simulink model "model"  (R2020b)
settings: Solver=VariableStepAuto  StartTime=0.0  StopTime=10.0  MaxStep=0.001  RelTol=1e-3
settings Model: Creator=Vrunda M Balgi  LastModifiedBy=Vrunda M Balgi

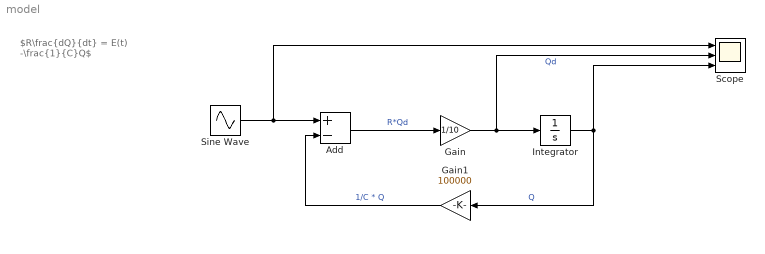
== system model ==
  note: $R\frac{dQ}{dt} = E(t) -\frac{1}{C}Q$
  Add : Sum  Inputs=+-
  Gain : Gain  Gain=1/10
  Gain1 : Gain  Gain=100000
  Integrator : Integrator
  Scope : Scope  NumInputPorts=3
  Sine Wave : Sin  Frequency=2*pi  SampleTime=0
  wires:
  Add/1 -> Gain/1  "R*Qd"
  Gain/1 -> Scope/2, Integrator/1  "Qd"
  Integrator/1 -> Scope/3, Gain1/1  "Q"
  Gain1/1 -> Add/2  "1/C * Q"
  Sine Wave/1 -> Scope/1, Add/1
